simulink model "Hexa_interface_harness"  (R2023a)
settings: Solver=ode4  StartTime=0.0  StopTime=200  FixedStep=0.01  RelTol=1e-3
PreLoadFcn:
  | load('Hexa_interface_harness_fmu_base.mat')
settings Model: Creator=danie  LastModifiedBy=danie

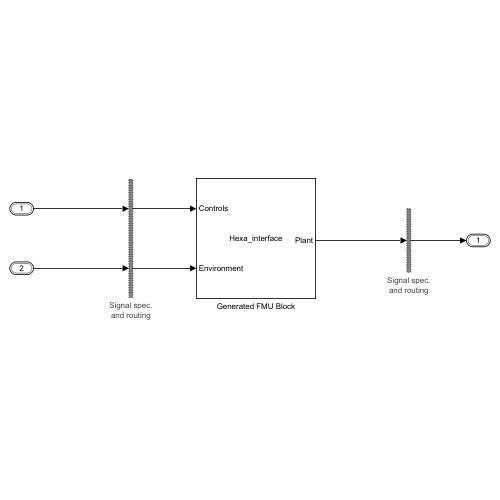
[thumbnail: Simulink's stored preview of the top-level diagram]
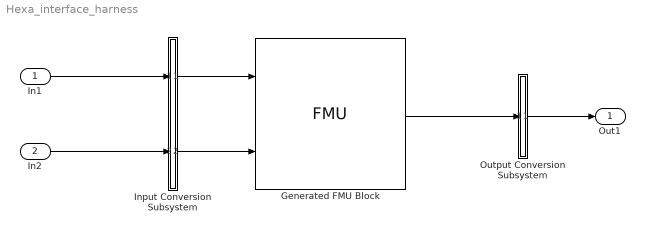
== system Hexa_interface_harness ==
  In1 : Inport  OutDataTypeStr=Bus: ControlsBusDef  PortDimensions=[1]  SampleTime=0.01  BusOutputAsStruct=on
  In2 : Inport  Port=2  OutDataTypeStr=Bus: EnvironmentBusDef  PortDimensions=[1]  SampleTime=0.01  BusOutputAsStruct=on
  Generated FMU Block : FMU  FMUName=Hexa_interface  FMUMode=CoSimulation  FMUSampleTime=0.01  FMUCreateBusObject=off  FMUCachedDialogLayout="{\"Geometry\":[1081,375,535,461],\"ParameterColumnsWidthConfig\":\"{\\\"columns\\\":[{\\\"name\\\":\\\"Parameter\\\",\\\"width\\\":144},{\\\"name\\\":\\\"Value\\\",\\\"width\\\":115},{\\\"name\\\":\\\"Unit\\\",\\\"width\\\":107},{\\\"name\\\":\\\"Description\\\",\\\"width\\\":149}]}\",\"InputColumnsWidthConfig\":\"{\\\"columns\\\":[{\\\"name\\\":\\\"Name\\\",\\\"width\\\":111},{\\\"name\\\":\\\"Visibility\\\",\\\"width\\\":60},{\\\"name\\\":\\\"Start\\\",\\\"width\\\":103},{\\\"name\\\":\\\"Unit\\\",\\\"width\\\":99},{\\\"name\\\":\\\"Bus Object\\\",\\\"width\\\":138}]}\",\"OutputColumnsWidthConfig\":\"{\\\"columns\\\":[{\\\"name\\\":\\\"Name\\\",\\\"width\\\":111},{\\\"name\\\":\\\"Visibility\\\",\\\"width\\\":60},{\\\"name\\\":\\\"Start\\\",\\\"width\\\":103},{\\\"name\\\":\\\"Unit\\\",\\\"width\\\":99},{\\\"name\\\":\\\"Bus Object\\\",\\\"width\\\":138}]}\"}"  HexaConstants=struct('Mass',1.8188,'Inertia',reshape([0.039375,0,0,0,0.040432,0,0,0,0.062148], [3,3]),'invallo',reshape([-105396.2901,105396.2901,0,-105396.2901,105396.2901,0,60856.8647,60856.8647,-121713.7293,60856.8647,60856.8647,-121713.7293,22151.09,22151.09,22143.0027,22151.09,22151.09,22143.0027,147579.693,147579.693,0,-147579.693,-147579.693,0,-85207.9073,85207.9073,170415.8146,85207.9073,-85207.9073,-170415.8146,200803.2129,-200803.2129,200803.2129,-200803.2129,200803.2129,-200803.2129], [6,6]),'kT',8.0082e-06)  mask(Hexa_interface [Co-Simulation, v2.0]){}
      mask Display:
      | disp('Hexa_interface');
      | port_label('output',1,'Plant');
      | port_label('input',1,'Controls');
      | port_label('input',2,'Environment');
  Input Conversion Subsystem : Subsystem  Tag=__SLT_ICS__  Description=|
      | Signal spec.
      | and routing
      settings: AttributesFormatString=%<Description>
  Output Conversion Subsystem : Subsystem  Tag=__SLT_OCS__  Description=|
      | Signal spec.
      | and routing
      settings: AttributesFormatString=%<Description>
  Out1 : Outport  OutDataTypeStr=Bus: PlantBusDef
  wires:
  In1/1 -> Input Conversion Subsystem/1(Inport_1)
  In2/1 -> Input Conversion Subsystem/2(Inport_2)
  Output Conversion Subsystem/1(Outport_1) -> Out1/1
  Input Conversion Subsystem/1(Outport_1) -> Generated FMU Block/1
  Input Conversion Subsystem/2(Outport_2) -> Generated FMU Block/2
  Generated FMU Block/1 -> Output Conversion Subsystem/1(Inport_1)

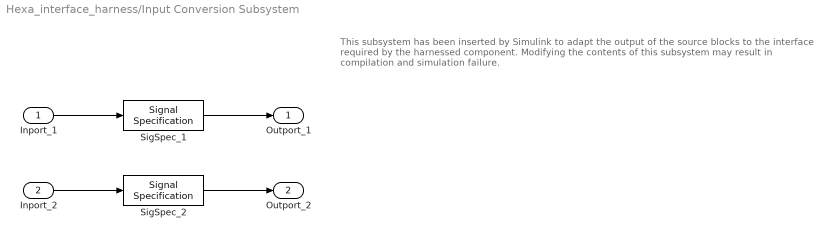
== system Hexa_interface_harness/Input Conversion Subsystem ==
  note: This subsystem has been inserted by Simulink to adapt the output of the source blocks to the interface required by the harnessed component.
      |  Modifying the contents of this subsystem may result in compilation and simulation failure.
  Inport_1 : Inport
  Inport_2 : Inport  Port=2
  SigSpec_1 : SignalSpecification  OutDataTypeStr=Bus: ControlsBusDef  Dimensions=[1]  SampleTime=0.01  BusOutputAsStruct=on
  SigSpec_2 : SignalSpecification  OutDataTypeStr=Bus: EnvironmentBusDef  Dimensions=[1]  SampleTime=0.01  BusOutputAsStruct=on
  Outport_1 : Outport
  Outport_2 : Outport  Port=2
  wires:
  SigSpec_1/1 -> Outport_1/1
  Inport_1/1 -> SigSpec_1/1
  SigSpec_2/1 -> Outport_2/1
  Inport_2/1 -> SigSpec_2/1

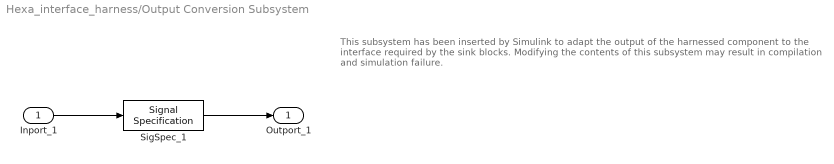
== system Hexa_interface_harness/Output Conversion Subsystem ==
  note: This subsystem has been inserted by Simulink to adapt the output of the harnessed component to the interface required by the sink blocks.
      |  Modifying the contents of this subsystem may result in compilation and simulation failure.
  Inport_1 : Inport
  SigSpec_1 : SignalSpecification  OutDataTypeStr=Bus: PlantBusDef  Dimensions=[1]  SampleTime=0.01  BusOutputAsStruct=on
  Outport_1 : Outport
  wires:
  Inport_1/1 -> SigSpec_1/1
  SigSpec_1/1 -> Outport_1/1
